simulink model "State_and_Output_Estimation_Simulink_Model"  (R2021a)
settings: Solver=VariableStepAuto  StartTime=0.0  StopTime=10.0  RelTol=1e-3
values from neighbouring files (symbols this model uses):
  A = [0, 1, 0, 0, 0, 0, 0, 0, 0, 0, 0, 0 ... (first row only)    [State_and_Output_Estimation_Matlab_Script.m]
  B = [0, 0, 0, 0 ... (first row only)    [State_and_Output_Estimation_Matlab_Script.m]
  C = [1, 0, 0, 0, 0, 0, 0, 0, 0, 0, 0, 0 ... (first row only)    [State_and_Output_Estimation_Matlab_Script.m]
  D = [0, 0, 0, 0 ... (first row only)    [State_and_Output_Estimation_Matlab_Script.m]
  q = 1e-3    (= 0.001)    [State_and_Output_Estimation_Matlab_Script.m]
  R = [1, 0, 0, 0, 0, 0, 0, 0, 0, 0, 0, 0 ... (first row only)    [State_and_Output_Estimation_Matlab_Script.m]
  Ts = 0.01    [State_and_Output_Estimation_Matlab_Script.m]
undefined symbols (not defined in the file or in its folder): Continuous, Time
libraries: simulink x24, ctrlSharedLib x1
settings Model: Creator=Vaibhav Bisht  LastModifiedBy=Vaibhav Bisht

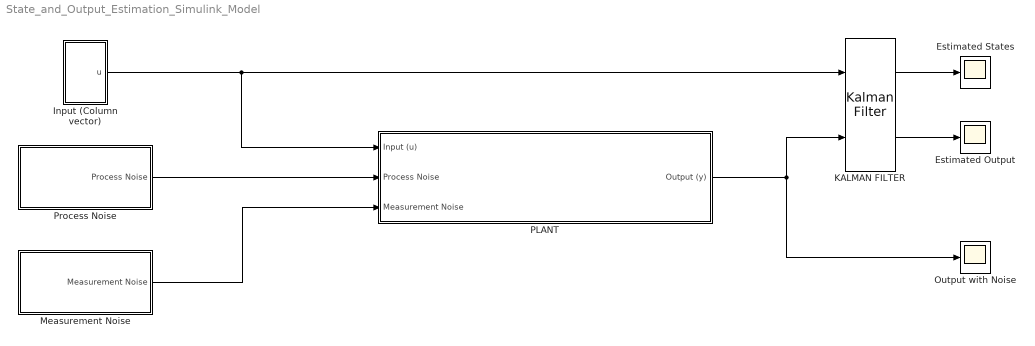
== system State_and_Output_Estimation_Simulink_Model ==
  Estimated Output : Scope
  Estimated States : Scope
  Input (Column vector) : Subsystem
  KALMAN FILTER : ctrlSharedLib/Kalman Filter  TimeDomain=Continuous-Time  UseCurrentEstimator=on  ModelSource=Individual A, B, C, D matrices  ModelSourceVariable=ss(0.95,1,1,0,1)  A=A  B=B  C=C  D=D  NumberOfStates=1  NumberOfInputs=1  NumberOfOutputs=1  InitialEstimateSource=Dialog  X0=[0 0 0 0 10 0 0 0 0 0 7 0]  P0=10  UseK=off  UseGH=off  NumberOfProcessNoiseInputs=1  G=1  TimeInvariantG=on  H=0  TimeInvariantH=on  Q=Q  TimeInvariantQ=on  R=R  TimeInvariantR=on  N=0  TimeInvariantN=on  AddInputPort=on  AddEnablePort=off  OutputEstimatedY=on  OutputP=off  Ts=-1
  Measurement Noise : Subsystem
  Output with Noise : Scope
  PLANT : Subsystem
  Process Noise : Subsystem
  wires:
  KALMAN FILTER/1 -> Estimated States/1
  KALMAN FILTER/2 -> Estimated Output/1
  PLANT/1(Output (y)) -> KALMAN FILTER/2, Output with Noise/1
  Process Noise/1(Process Noise) -> PLANT/2(Process Noise)
  Measurement Noise/1(Measurement Noise) -> PLANT/3(Measurement Noise)
  Input (Column vector)/1(u) -> PLANT/1(Input (u)), KALMAN FILTER/1

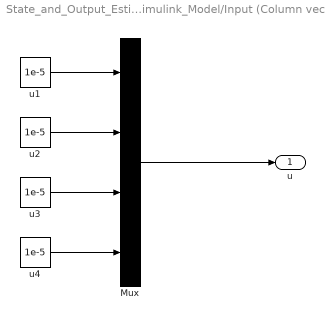
== system State_and_Output_Estimation_Simulink_Model/Input (Column vector) ==
  Mux : Mux
  u{1..4} (4 alike) : Constant  Value=1e-5
  u : Outport
  wires:
  u3/1 -> Mux/3
  u2/1 -> Mux/2
  u1/1 -> Mux/1
  u4/1 -> Mux/4
  Mux/1 -> u/1

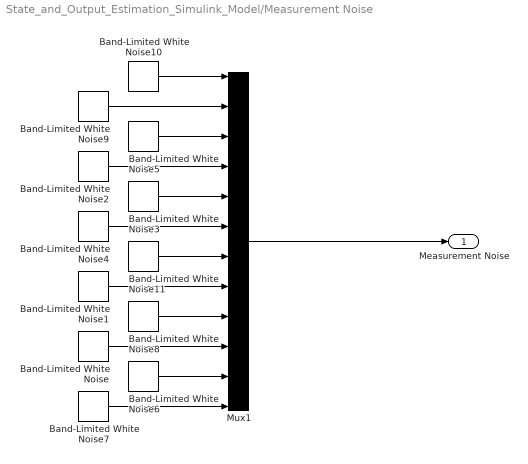
== system State_and_Output_Estimation_Simulink_Model/Measurement Noise ==
  Band-Limited White Noise{,1..11} (12 alike) : simulink/Sources/Band-Limited White Noise  Cov=q*Ts  Ts=Ts  seed=[23341]
  Mux1 : Mux  Inputs=12
  Measurement Noise : Outport
  wires:
  Mux1/1 -> Measurement Noise/1
  Band-Limited White Noise2/1 -> Mux1/4
  Band-Limited White Noise8/1 -> Mux1/9
  Band-Limited White Noise10/1 -> Mux1/1
  Band-Limited White Noise1/1 -> Mux1/8
  Band-Limited White Noise7/1 -> Mux1/12
  Band-Limited White Noise11/1 -> Mux1/7
  Band-Limited White Noise/1 -> Mux1/10
  Band-Limited White Noise4/1 -> Mux1/6
  Band-Limited White Noise9/1 -> Mux1/2
  Band-Limited White Noise5/1 -> Mux1/3
  Band-Limited White Noise3/1 -> Mux1/5
  Band-Limited White Noise6/1 -> Mux1/11

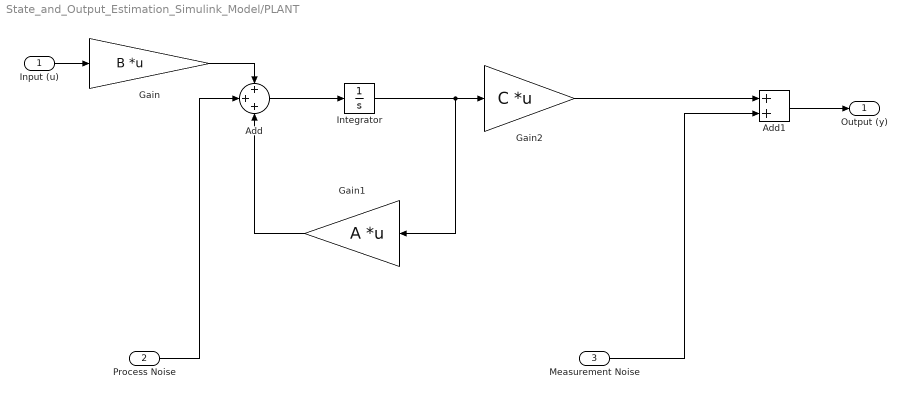
== system State_and_Output_Estimation_Simulink_Model/PLANT ==
  Input (u) : Inport
  Process Noise : Inport  Port=2
  Measurement Noise : Inport  Port=3
  Add : Sum  Inputs=+++
  Add1 : Sum
  Gain : Gain  Gain=B  Multiplication=Matrix(K*u) (u vector)
  Gain1 : Gain  Gain=A  Multiplication=Matrix(K*u) (u vector)
  Gain2 : Gain  Gain=C  Multiplication=Matrix(K*u) (u vector)
  Integrator : Integrator  InitialCondition=[0 0 0 0 10 0 0 0 0 0 7 0]
  Output (y) : Outport
  wires:
  Add/1 -> Integrator/1
  Gain2/1 -> Add1/1
  Gain1/1 -> Add/3
  Integrator/1 -> Gain2/1, Gain1/1
  Gain/1 -> Add/1
  Input (u)/1 -> Gain/1
  Measurement Noise/1 -> Add1/2
  Process Noise/1 -> Add/2
  Add1/1 -> Output (y)/1

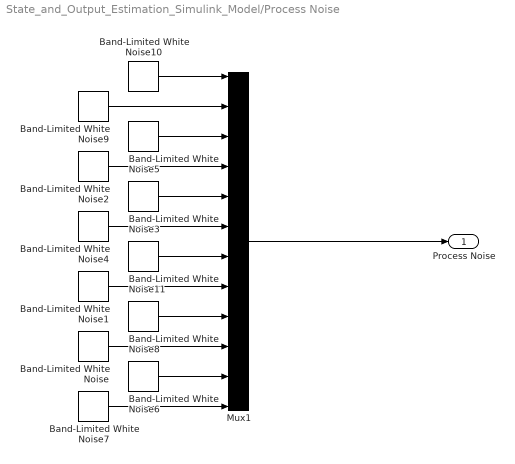
== system State_and_Output_Estimation_Simulink_Model/Process Noise ==
  Band-Limited White Noise{,1..11} (12 alike) : simulink/Sources/Band-Limited White Noise  Cov=q*Ts  Ts=Ts  seed=[23341]
  Mux1 : Mux  Inputs=12
  Process Noise : Outport
  wires:
  Band-Limited White Noise6/1 -> Mux1/11
  Band-Limited White Noise3/1 -> Mux1/5
  Band-Limited White Noise5/1 -> Mux1/3
  Band-Limited White Noise9/1 -> Mux1/2
  Band-Limited White Noise4/1 -> Mux1/6
  Band-Limited White Noise/1 -> Mux1/10
  Band-Limited White Noise11/1 -> Mux1/7
  Band-Limited White Noise7/1 -> Mux1/12
  Band-Limited White Noise1/1 -> Mux1/8
  Band-Limited White Noise10/1 -> Mux1/1
  Band-Limited White Noise8/1 -> Mux1/9
  Band-Limited White Noise2/1 -> Mux1/4
  Mux1/1 -> Process Noise/1
